simulink model "grafica1pam"  (R2019a)
settings: Solver=VariableStepAuto  StartTime=0.0  StopTime=0.3  RelTol=1e-3
libraries: dsparch4 x1
settings Model: NumberOfSteps=3  Creator=JORGE  LastModifiedBy=JORGE
settings ModelReferenceCC: ModelReferenceNumInstancesAllowed=Single

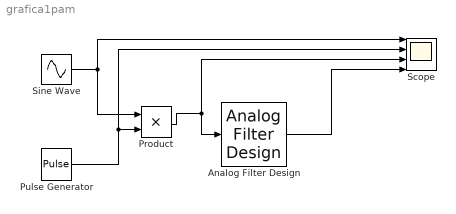
== system grafica1pam ==
  Analog Filter Design : dsparch4/Analog Filter Design  method=Butterworth  filttype=Lowpass  N=3  Wlo=2*pi*20  Whi=80  Rp=2  Rs=40
  Product : Product
  Pulse Generator : DiscretePulseGenerator  PulseType=Time based  Period=0.025  PulseWidth=5
  Scope : Scope  NumInputPorts=4
  Sine Wave : Sin  Frequency=2*pi*20  Phase=pi/2  SampleTime=0.001
  wires:
  Sine Wave/1 -> Scope/1, Product/1
  Pulse Generator/1 -> Scope/2, Product/2
  Product/1 -> Scope/3, Analog Filter Design/1
  Analog Filter Design/1 -> Scope/4
